simulink model "remaining_mass_calculator"  (R2020b)
settings: Solver=VariableStepAuto  StartTime=0.0  StopTime=10.0  RelTol=1e-3
undefined symbols (not defined in the file): P_mc_dry_mass_rocket, P_mc_fuel_rocket, P_mc_wet_mass_rocket
settings Model: Creator=wizard  LastModifiedBy=wizard

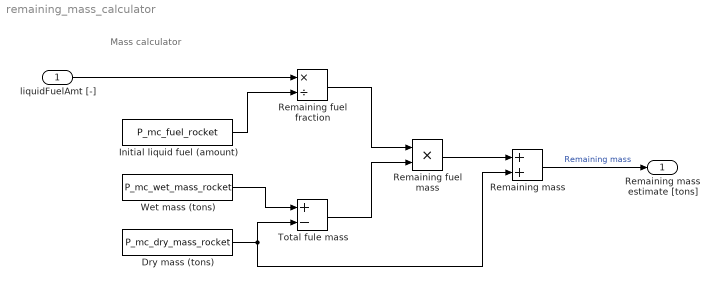
== system remaining_mass_calculator ==
  note: Mass calculator
  liquidFuelAmt [-] : Inport
  Dry mass (tons) : Constant  Value=P_mc_dry_mass_rocket  OutDataTypeStr=double
  Initial liquid fuel (amount) : Constant  Value=P_mc_fuel_rocket  OutDataTypeStr=double
  Remaining fuel fraction : Product  Inputs=*/
  Remaining fuel mass : Product  Inputs=**
  Remaining mass : Sum
  Total fule mass : Sum  Inputs=+-
  Wet mass (tons) : Constant  Value=P_mc_wet_mass_rocket  OutDataTypeStr=double
  Remaining mass estimate [tons] : Outport
  wires:
  Initial liquid fuel (amount)/1 -> Remaining fuel fraction/2
  Dry mass (tons)/1 -> Remaining mass/2, Total fule mass/2
  Remaining fuel mass/1 -> Remaining mass/1
  Total fule mass/1 -> Remaining fuel mass/2
  liquidFuelAmt [-]/1 -> Remaining fuel fraction/1
  Wet mass (tons)/1 -> Total fule mass/1
  Remaining mass/1 -> Remaining mass estimate [tons]/1  "Remaining mass"
  Remaining fuel fraction/1 -> Remaining fuel mass/1
